simulink model "Supersonic_SAS"  (R2020a)
settings: Solver=VariableStepAuto  StartTime=0.0  StopTime=10.0  RelTol=1e-3
values from neighbouring files (symbols this model uses):
  A = [(Y_b/u_o) (Y_p/u_o) -(1 - (Y_r/u_o)) (g/u_o) ; L_b L_p L_r 0 ; N_b N_p N_r 0 ; 0 1 0 0]    [Approach_1.m]    (also in Supersonic.m = [Y_B/u0 Y_p/u0 -(1-(Y_r/u0)) g/u0; L_B L_p L_r 0; N_B N_p N_)
  B = [0 Y_del_r/u_o ; L_del_a L_del_r ; N_del_a N_del_r ; 0 0]    [Approach_1.m]    (also in Supersonic.m = [0 Y_delta_r/u0; L_delta_a L_delta_r; N_delta_a N_delta_r; 0)
  C = [1 0 0 0 ; 0 1 0 0 ; 0 0 1 0 ; 0 0 0 1]    [Approach_1.m]    (also in Supersonic.m = [1 0 0 0; 0 1 0 0; 0 0 1 0; 0 0 0 1])
  D = [0 0 ; 0 0 ; 0 0 ; 0 0]    [Approach_1.m]    (also in Supersonic.m = [0 0; 0 0; 0 0; 0 0])
settings Model: Creator=AHSAN  LastModifiedBy=AHSAN

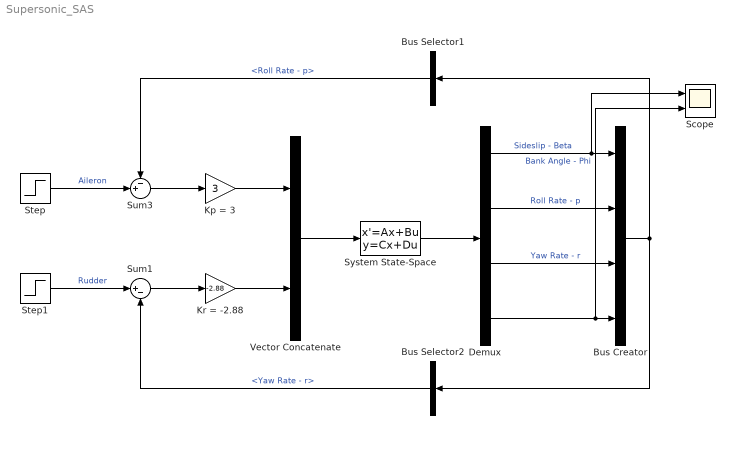
== system Supersonic_SAS ==
  Bus Creator : BusCreator  Inputs=4
  Bus Selector1 : BusSelector  OutputSignals=Roll Rate - p
  Bus Selector2 : BusSelector  OutputSignals=Yaw Rate - r
  Demux : Demux
  Kp = 3 : Gain  Gain=3
  Kr = -2.88 : Gain  Gain=-2.88
  Scope : Scope  NumInputPorts=2
  Step : Step  Time=0  SampleTime=0
  Step1 : Step  SampleTime=0
  Sum1 : Sum  Inputs=|+-
  Sum3 : Sum  Inputs=-+|
  System State-Space : StateSpace  A=A  B=B  C=C  D=D  InitialCondition=0
  Vector Concatenate : Concatenate
  wires:
  Kp = 3/1 -> Vector Concatenate/1
  Bus Selector1/1 -> Sum3/1  "<Roll Rate - p>"
  System State-Space/1 -> Demux/1
  Demux/2 -> Bus Creator/2  "Roll Rate - p"
  Bus Creator/1 -> Bus Selector2/1, Bus Selector1/1
  Demux/1 -> Bus Creator/1, Scope/1  "Sideslip - Beta"
  Vector Concatenate/1 -> System State-Space/1
  Sum3/1 -> Kp = 3/1
  Demux/4 -> Bus Creator/4, Scope/2  "Bank Angle - Phi"
  Demux/3 -> Bus Creator/3  "Yaw Rate - r"
  Step/1 -> Sum3/2  "Aileron"
  Bus Selector2/1 -> Sum1/2  "<Yaw Rate - r>"
  Kr = -2.88/1 -> Vector Concatenate/2
  Sum1/1 -> Kr = -2.88/1
  Step1/1 -> Sum1/1  "Rudder"
